simulink model "T_TEM_OCV"  (R2015a)
settings: Solver=ode3  StartTime=0.0  StopTime=6  FixedStep=1  RelTol=1e-3
values from neighbouring files (symbols this model uses):
  I = 0    [TEM_OCV.m]
  T_c = 273+25    (= 298)    [TEM_OCV.m]
libraries: LU_TEG x2
settings Model: Creator=lansong7  LastModifiedBy=lansong7

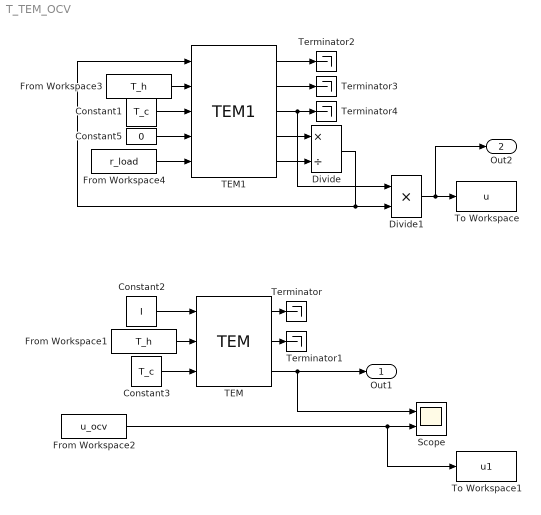
== system T_TEM_OCV ==
  Constant1 : Constant  Value=T_c
  Constant2 : Constant  Value=I
  Constant3 : Constant  Value=T_c
  Constant5 : Constant  Value=0
  Divide : Product  Inputs=*/
  Divide1 : Product  Inputs=**
  From Workspace1 : FromWorkspace  VariableName=T_h  SampleTime=0
  From Workspace2 : FromWorkspace  VariableName=u_ocv  SampleTime=0
  From Workspace3 : FromWorkspace  VariableName=T_h  SampleTime=0
  From Workspace4 : FromWorkspace  VariableName=r_load  SampleTime=0
  Scope : Scope  NumInputPorts=2
      settings: TimeRange=159  YMin=300~0  YMax=380~7
  TEM : LU_TEG/TEM  l=l  l_cw=l_cw  f=f  a=a  n=n  Tune_tr=Tune_tr  Tune_er=Tune_er  ct1=ct1  ct2=ct2
  TEM1 : LU_TEG/TEM1  l=l  l_cw=l_cw  f=f  a=a  n=n  Tune_tr=Tune_tr  Tune_er=Tune_er  ct1=ct1  ct2=ct2  M=M
  Terminator{,1..4} (5 alike) : Terminator
  To Workspace : ToWorkspace  VariableName=u  SaveFormat=Structure With Time  SampleTime=-1
  To Workspace1 : ToWorkspace  VariableName=u1  SaveFormat=Structure With Time  SampleTime=-1
  Out1 : Outport
  Out2 : Outport  Port=2
  wires:
  Constant2/1 -> TEM/1
  TEM/1 -> Terminator/1
  From Workspace2/1 -> To Workspace1/1, Scope/2
  From Workspace1/1 -> TEM/2
  Constant3/1 -> TEM/3
  TEM/2 -> Terminator1/1
  TEM/3 -> Scope/1, Out1/1
  From Workspace3/1 -> TEM1/2
  Constant1/1 -> TEM1/3
  From Workspace4/1 -> TEM1/5
  Constant5/1 -> TEM1/4
  TEM1/1 -> Terminator2/1
  TEM1/2 -> Terminator3/1
  TEM1/3 -> Divide1/1, Terminator4/1
  TEM1/5 -> Divide/2
  TEM1/4 -> Divide/1
  Divide/1 -> TEM1/1, Divide1/2
  Divide1/1 -> Out2/1, To Workspace/1
